simulink model "k1modalitmx"  (Simulink 8.6)
settings: Solver=VariableStepAuto  StartTime=0.0  StopTime=10.0  RelTol=1e-3
libraries: cdsIPCx x30, cdsAdcx0 x1, cdsAdcx1 x1, VISMODAL_MASTER x1, cdsParameters x1
settings Model: Creator=controls  LastModifiedBy=controls
settings DataIOCC: SaveFormat=Dataset  SignalLoggingSaveFormat=Dataset
settings OptimizationCC: ExpressionDepthLimit=128
settings DebuggingCC: UnderspecifiedInitializationDetection=Simplified  MergeDetectMultiDrivingBlocksExec=error  SolverPrmCheckMsg=none  FcnCallInpInsideContextMsg=EnableAllAsError  StateNameClashWarn=none
settings HardwareCC: ProdBitPerPointer=64  ProdLargestAtomicFloat=Float  ProdIntDivRoundTo=Zero  ProdEndianess=LittleEndian  ProdWordSize=64  ProdHWDeviceType=Intel->x86-64 (Windows64)
settings GRTTargetCC: GeneratePreprocessorConditionals=Use local settings  CombineOutputUpdateFcns=on  GRTInterface=off
settings ConfigComp: CovModelRefEnable=off

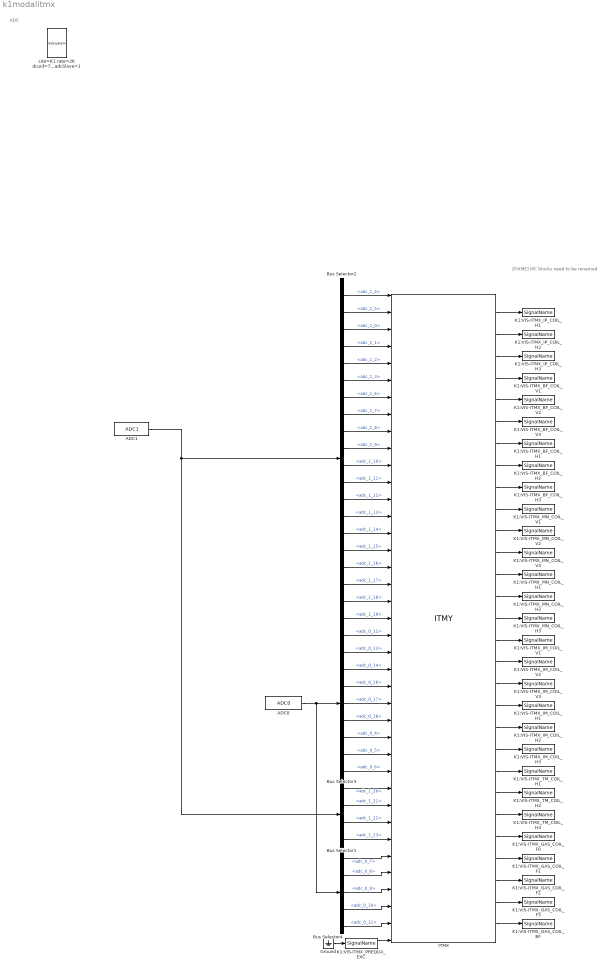
== system k1modalitmx ==
  note: ADC
  note: [FIXME] IPC blocks need to be renamed
  ADC0 : cdsAdcx0/ADC0  Tag=cdsAdc  Description=|
      | type-GSC_16AI64SSA
      | card_num=0
      settings: AttributesFormatString=%<Description>\n%<Tag>
  ADC1 : cdsAdcx1/ADC1  Tag=cdsAdc  Description=|
      | type-GSC_16AI64SSA
      | card_num=1
      settings: AttributesFormatString=%<Description>\n%<Tag>
  Bus Selector1 : BusSelector  OutputSignals=adc_1_20,adc_1_21,adc_1_22,adc_1_23
  Bus Selector2 : BusSelector  OutputSignals=adc_1_4,adc_1_5,adc_1_0,adc_1_1,adc_1_2,adc_1_3,adc_1_6,adc_1_7,adc_1_8,adc_1_9,adc_1_10,adc_1_11,adc_1_12,adc_1_13,adc_1_14,adc_1_15,adc_1_16,adc_1_17,adc_1_18,adc_1_19
  Bus Selector3 : BusSelector  OutputSignals=adc_0_12,adc_0_13,adc_0_14,adc_0_16,adc_0_17,adc_0_18,adc_0_4,adc_0_5,adc_0_6
  Bus Selector4 : BusSelector  OutputSignals=adc_0_7,adc_0_8,adc_0_9,adc_0_10,adc_0_11
  Ground : Ground
  ITMX : VISMODAL_MASTER/ITMY
  K1:VIS-ITMX_BF_COIL_H1 : cdsIPCx/SignalName  Tag=cdsIPCx_SHMEM  Description=Inter-Process Communication via Shared memory.
      settings: AttributesFormatString=%<Tag>
  K1:VIS-ITMX_BF_COIL_H2 : cdsIPCx/SignalName  Tag=cdsIPCx_SHMEM  Description=Inter-Process Communication via Shared memory.
      settings: AttributesFormatString=%<Tag>
  K1:VIS-ITMX_BF_COIL_H3 : cdsIPCx/SignalName  Tag=cdsIPCx_SHMEM  Description=Inter-Process Communication via Shared memory.
      settings: AttributesFormatString=%<Tag>
  K1:VIS-ITMX_BF_COIL_V1 : cdsIPCx/SignalName  Tag=cdsIPCx_SHMEM  Description=Inter-Process Communication via Shared memory.
      settings: AttributesFormatString=%<Tag>
  K1:VIS-ITMX_BF_COIL_V2 : cdsIPCx/SignalName  Tag=cdsIPCx_SHMEM  Description=Inter-Process Communication via Shared memory.
      settings: AttributesFormatString=%<Tag>
  K1:VIS-ITMX_BF_COIL_V3 : cdsIPCx/SignalName  Tag=cdsIPCx_SHMEM  Description=Inter-Process Communication via Shared memory.
      settings: AttributesFormatString=%<Tag>
  K1:VIS-ITMX_GAS_COIL_BF : cdsIPCx/SignalName  Tag=cdsIPCx_SHMEM  Description=Inter-Process Communication via Shared memory.
      settings: AttributesFormatString=%<Tag>
  K1:VIS-ITMX_GAS_COIL_F{0..3} (4 alike) : cdsIPCx/SignalName  Tag=cdsIPCx_SHMEM  Description=Inter-Process Communication via Shared memory.
      settings: AttributesFormatString=%<Tag>
  K1:VIS-ITMX_IM_COIL_H1 : cdsIPCx/SignalName  Tag=cdsIPCx_SHMEM  Description=Inter-Process Communication via Shared memory.
      settings: AttributesFormatString=%<Tag>
  K1:VIS-ITMX_IM_COIL_H2 : cdsIPCx/SignalName  Tag=cdsIPCx_SHMEM  Description=Inter-Process Communication via Shared memory.
      settings: AttributesFormatString=%<Tag>
  K1:VIS-ITMX_IM_COIL_H3 : cdsIPCx/SignalName  Tag=cdsIPCx_SHMEM  Description=Inter-Process Communication via Shared memory.
      settings: AttributesFormatString=%<Tag>
  K1:VIS-ITMX_IM_COIL_V1 : cdsIPCx/SignalName  Tag=cdsIPCx_SHMEM  Description=Inter-Process Communication via Shared memory.
      settings: AttributesFormatString=%<Tag>
  K1:VIS-ITMX_IM_COIL_V2 : cdsIPCx/SignalName  Tag=cdsIPCx_SHMEM  Description=Inter-Process Communication via Shared memory.
      settings: AttributesFormatString=%<Tag>
  K1:VIS-ITMX_IM_COIL_V3 : cdsIPCx/SignalName  Tag=cdsIPCx_SHMEM  Description=Inter-Process Communication via Shared memory.
      settings: AttributesFormatString=%<Tag>
  K1:VIS-ITMX_IP_COIL_H1 : cdsIPCx/SignalName  Tag=cdsIPCx_SHMEM  Description=Inter-Process Communication via Shared memory.
      settings: AttributesFormatString=%<Tag>
  K1:VIS-ITMX_IP_COIL_H2 : cdsIPCx/SignalName  Tag=cdsIPCx_SHMEM  Description=Inter-Process Communication via Shared memory.
      settings: AttributesFormatString=%<Tag>
  K1:VIS-ITMX_IP_COIL_H3 : cdsIPCx/SignalName  Tag=cdsIPCx_SHMEM  Description=Inter-Process Communication via Shared memory.
      settings: AttributesFormatString=%<Tag>
  K1:VIS-ITMX_MN_COIL_H1 : cdsIPCx/SignalName  Tag=cdsIPCx_SHMEM  Description=Inter-Process Communication via Shared memory.
      settings: AttributesFormatString=%<Tag>
  K1:VIS-ITMX_MN_COIL_H2 : cdsIPCx/SignalName  Tag=cdsIPCx_SHMEM  Description=Inter-Process Communication via Shared memory.
      settings: AttributesFormatString=%<Tag>
  K1:VIS-ITMX_MN_COIL_H3 : cdsIPCx/SignalName  Tag=cdsIPCx_SHMEM  Description=Inter-Process Communication via Shared memory.
      settings: AttributesFormatString=%<Tag>
  K1:VIS-ITMX_MN_COIL_V1 : cdsIPCx/SignalName  Tag=cdsIPCx_SHMEM  Description=Inter-Process Communication via Shared memory.
      settings: AttributesFormatString=%<Tag>
  K1:VIS-ITMX_MN_COIL_V2 : cdsIPCx/SignalName  Tag=cdsIPCx_SHMEM  Description=Inter-Process Communication via Shared memory.
      settings: AttributesFormatString=%<Tag>
  K1:VIS-ITMX_MN_COIL_V3 : cdsIPCx/SignalName  Tag=cdsIPCx_SHMEM  Description=Inter-Process Communication via Shared memory.
      settings: AttributesFormatString=%<Tag>
  K1:VIS-ITMX_PREQUA_EXC : cdsIPCx/SignalName  Tag=cdsIPCx_SHMEM  Description=Inter-Process Communication via Shared memory.
      settings: AttributesFormatString=%<Tag>
  K1:VIS-ITMX_TM_COIL_H1 : cdsIPCx/SignalName  Tag=cdsIPCx_SHMEM  Description=Inter-Process Communication via Shared memory.
      settings: AttributesFormatString=%<Tag>
  K1:VIS-ITMX_TM_COIL_H2 : cdsIPCx/SignalName  Tag=cdsIPCx_SHMEM  Description=Inter-Process Communication via Shared memory.
      settings: AttributesFormatString=%<Tag>
  K1:VIS-ITMX_TM_COIL_H3 : cdsIPCx/SignalName  Tag=cdsIPCx_SHMEM  Description=Inter-Process Communication via Shared memory.
      settings: AttributesFormatString=%<Tag>
  site=K1 rate=2K dcuid=70 host=k1ix1 specific_cpu=4 adcSlave=1 : cdsParameters/Subsystem  Tag=cdsParameters  Description=|
      | Purpose:                                                                                                                                                                                                                                
      | Provide system parameters to the FE code generator to properly configure the generated EPICS names, rep rate of the FE controller, and the Data Acquisition node ID for proper storage of data from this FE controller.                 
      |                                                                                                                                                                                                                                         
      | Useage:                                                                                                                                                                                                                                 
      | The part NAME field is used to identify the FE parameters. It must be of the form:                                                                                                                                                      
      | site=                                                                                                                                                                                                                                   
      | rate=                                                                                                                                                                                                                                   
      | dcuid=                                                                                                                                                                                                                                  
      |                                                                                                                                                                                                                                         
      | Where:                                                                                                                                                                                                                                  
      | site= argument may be H1, H2, L1, M1, G1, either as a single argument or multiple, for example site=H1,H2. These are the only names allowed. These will become the first two characters of all EPICS and signal names (for example G1:).
      |                                                                                                                                                                                                                                         
      | rate= may be 2K, 16K, 32K, or 64K                                                                                                                                                                                                       
      |                                                                                                                                                                                                                                         
      | dcuid= is site specific ie it must be unique at each site.
      settings: AttributesFormatString=%<Tag>
  wires:
  ITMX/10 -> K1:VIS-ITMX_MN_COIL_V1/1
  ITMX/11 -> K1:VIS-ITMX_MN_COIL_V2/1
  ITMX/12 -> K1:VIS-ITMX_MN_COIL_V3/1
  ITMX/13 -> K1:VIS-ITMX_MN_COIL_H1/1
  ITMX/14 -> K1:VIS-ITMX_MN_COIL_H2/1
  ITMX/15 -> K1:VIS-ITMX_MN_COIL_H3/1
  ITMX/16 -> K1:VIS-ITMX_IM_COIL_V1/1
  ITMX/17 -> K1:VIS-ITMX_IM_COIL_V2/1
  ITMX/18 -> K1:VIS-ITMX_IM_COIL_V3/1
  ITMX/19 -> K1:VIS-ITMX_IM_COIL_H1/1
  ITMX/20 -> K1:VIS-ITMX_IM_COIL_H2/1
  ITMX/21 -> K1:VIS-ITMX_IM_COIL_H3/1
  ITMX/22 -> K1:VIS-ITMX_TM_COIL_H1/1
  ITMX/23 -> K1:VIS-ITMX_TM_COIL_H2/1
  ITMX/24 -> K1:VIS-ITMX_TM_COIL_H3/1
  ITMX/1 -> K1:VIS-ITMX_IP_COIL_H1/1
  ITMX/2 -> K1:VIS-ITMX_IP_COIL_H2/1
  ITMX/3 -> K1:VIS-ITMX_IP_COIL_H3/1
  ITMX/4 -> K1:VIS-ITMX_BF_COIL_V1/1
  ITMX/5 -> K1:VIS-ITMX_BF_COIL_V2/1
  ITMX/6 -> K1:VIS-ITMX_BF_COIL_V3/1
  ITMX/7 -> K1:VIS-ITMX_BF_COIL_H1/1
  ITMX/8 -> K1:VIS-ITMX_BF_COIL_H2/1
  ITMX/9 -> K1:VIS-ITMX_BF_COIL_H3/1
  ADC1/1 -> Bus Selector1/1, Bus Selector2/1
  Bus Selector2/1 -> ITMX/1  "<adc_1_4>"
  Bus Selector2/2 -> ITMX/2  "<adc_1_5>"
  Bus Selector2/3 -> ITMX/3  "<adc_1_0>"
  Bus Selector2/4 -> ITMX/4  "<adc_1_1>"
  Bus Selector2/5 -> ITMX/5  "<adc_1_2>"
  Bus Selector2/6 -> ITMX/6  "<adc_1_3>"
  Bus Selector2/7 -> ITMX/7  "<adc_1_6>"
  Bus Selector2/8 -> ITMX/8  "<adc_1_7>"
  Bus Selector2/9 -> ITMX/9  "<adc_1_8>"
  Bus Selector2/10 -> ITMX/10  "<adc_1_9>"
  Bus Selector2/11 -> ITMX/11  "<adc_1_10>"
  Bus Selector2/12 -> ITMX/12  "<adc_1_11>"
  Bus Selector2/13 -> ITMX/13  "<adc_1_12>"
  Bus Selector2/14 -> ITMX/14  "<adc_1_13>"
  Bus Selector2/15 -> ITMX/15  "<adc_1_14>"
  Bus Selector2/16 -> ITMX/16  "<adc_1_15>"
  Bus Selector2/17 -> ITMX/17  "<adc_1_16>"
  Bus Selector2/18 -> ITMX/18  "<adc_1_17>"
  Bus Selector2/19 -> ITMX/19  "<adc_1_18>"
  Bus Selector2/20 -> ITMX/20  "<adc_1_19>"
  ADC0/1 -> Bus Selector4/1, Bus Selector3/1
  Bus Selector3/1 -> ITMX/21  "<adc_0_12>"
  Bus Selector3/2 -> ITMX/22  "<adc_0_13>"
  Bus Selector3/3 -> ITMX/23  "<adc_0_14>"
  Bus Selector3/4 -> ITMX/24  "<adc_0_16>"
  Bus Selector3/5 -> ITMX/25  "<adc_0_17>"
  Bus Selector3/6 -> ITMX/26  "<adc_0_18>"
  Bus Selector3/7 -> ITMX/27  "<adc_0_4>"
  Bus Selector3/8 -> ITMX/28  "<adc_0_5>"
  Bus Selector3/9 -> ITMX/29  "<adc_0_6>"
  Bus Selector1/1 -> ITMX/30  "<adc_1_20>"
  Bus Selector1/2 -> ITMX/31  "<adc_1_21>"
  Bus Selector1/3 -> ITMX/32  "<adc_1_22>"
  Bus Selector1/4 -> ITMX/33  "<adc_1_23>"
  ITMX/25 -> K1:VIS-ITMX_GAS_COIL_F0/1
  ITMX/26 -> K1:VIS-ITMX_GAS_COIL_F1/1
  ITMX/27 -> K1:VIS-ITMX_GAS_COIL_F2/1
  ITMX/28 -> K1:VIS-ITMX_GAS_COIL_F3/1
  ITMX/29 -> K1:VIS-ITMX_GAS_COIL_BF/1
  Bus Selector4/1 -> ITMX/34  "<adc_0_7>"
  Bus Selector4/2 -> ITMX/35  "<adc_0_8>"
  Bus Selector4/3 -> ITMX/36  "<adc_0_9>"
  Bus Selector4/4 -> ITMX/37  "<adc_0_10>"
  Bus Selector4/5 -> ITMX/38  "<adc_0_11>"
  K1:VIS-ITMX_PREQUA_EXC/1 -> ITMX/39
  Ground/1 -> K1:VIS-ITMX_PREQUA_EXC/1
